simulink model "gm_parallel_prediction_and_cost_function_6phase"  (R2022a)
settings: Solver=FixedStepDiscrete  StartTime=0.0  StopTime=10.0  RelTol=1e-3
undefined symbols (not defined in the file or in its folder): f_c, L_d, L_q, L_x, L_y, p, psi_pm, R_ph
libraries: hdlmdlgenlib x2
(part 3 of 8)

== system gm_parallel_prediction_and_cost_function_6phase/Prediction_and_cost_function/Detect Rise Positive ==
  note: Edge
  note: U(k)
  U : Inport  OutDataTypeStr=boolean  SampleTime=1e-08
  Delay Input1 : UnitDelay  Description=Store in Global RAM  DisableCoverage=on  InitialCondition=vinit  SampleTime=-1  HasFrameUpgradeWarning=on
  FixPt Relational Operator : RelationalOperator  Operator=>  OutDataTypeStr=boolean  ZeroCross=off  InputSameDT=off
  Positive : Subsystem  mask(Compare To Zero){relop=>, OutDataTypeStr=boolean, ZeroCross=off}
      mask prompts: relop "Simulink:masks:Operator_MP"; OutDataTypeStr "Simulink:masks:OutputDataType_MP"; ZeroCross "Simulink:masks:EnableZerocrossingDetection_MP"
      mask help: Simulink:masks:CompareToZero_MD
      mask init:
      | OutDataTypeStr = 'boolean';
      | ZeroCross = 'off';
      | blkName = 'parallel_prediction_and_cost_function_6phase/Prediction_and_cost_function/Detect Rise\nPositive/Positive';
      | relop = '>';
      | setValue = 'boolean';
      mask TypeOptions relop: == | ~= | < | <= | >= | >
      mask TypeOptions OutDataTypeStr: Simulink:masks:uint8 | Simulink:masks:boolean
      mask Callback ZeroCross: sl('zeroCrossEnable', gcbh);
      mask Display: disp([relop,' 0'])
  Y : Outport  SampleTime=1e-08
  wires:
  Delay Input1/1 -> FixPt Relational Operator/2
  FixPt Relational Operator/1 -> Y/1
  Positive/1(y) -> FixPt Relational Operator/1, Delay Input1/1
  U/1 -> Positive/1(u)

== system gm_parallel_prediction_and_cost_function_6phase/Prediction_and_cost_function/Detect Rise Positive1 ==
  note: Edge
  note: U(k)
  U : Inport  OutDataTypeStr=boolean  SampleTime=1e-08
  Delay Input1 : UnitDelay  Description=Store in Global RAM  DisableCoverage=on  InitialCondition=vinit  SampleTime=-1  HasFrameUpgradeWarning=on
  FixPt Relational Operator : RelationalOperator  Operator=>  OutDataTypeStr=boolean  ZeroCross=off  InputSameDT=off
  Positive : Subsystem  mask(Compare To Zero){relop=>, OutDataTypeStr=boolean, ZeroCross=off}
      mask prompts: relop "Simulink:masks:Operator_MP"; OutDataTypeStr "Simulink:masks:OutputDataType_MP"; ZeroCross "Simulink:masks:EnableZerocrossingDetection_MP"
      mask help: Simulink:masks:CompareToZero_MD
      mask init:
      | OutDataTypeStr = 'boolean';
      | ZeroCross = 'off';
      | blkName = 'parallel_prediction_and_cost_function_6phase/Prediction_and_cost_function/Detect Rise\nPositive1/Positive';
      | relop = '>';
      | setValue = 'boolean';
      mask TypeOptions relop: == | ~= | < | <= | >= | >
      mask TypeOptions OutDataTypeStr: Simulink:masks:uint8 | Simulink:masks:boolean
      mask Callback ZeroCross: sl('zeroCrossEnable', gcbh);
      mask Display: disp([relop,' 0'])
  Y : Outport  SampleTime=1e-08
  wires:
  Delay Input1/1 -> FixPt Relational Operator/2
  FixPt Relational Operator/1 -> Y/1
  Positive/1(y) -> FixPt Relational Operator/1, Delay Input1/1
  U/1 -> Positive/1(u)

== system gm_parallel_prediction_and_cost_function_6phase/Prediction_and_cost_function/Detect Rise Positive2 ==
  note: Edge
  note: U(k)
  U : Inport  OutDataTypeStr=boolean  SampleTime=1e-08
  Delay Input1 : UnitDelay  Description=Store in Global RAM  DisableCoverage=on  InitialCondition=vinit  SampleTime=-1  HasFrameUpgradeWarning=on
  FixPt Relational Operator : RelationalOperator  Operator=>  OutDataTypeStr=boolean  ZeroCross=off  InputSameDT=off
  Positive : Subsystem  mask(Compare To Zero){relop=>, OutDataTypeStr=boolean, ZeroCross=off}
      mask prompts: relop "Simulink:masks:Operator_MP"; OutDataTypeStr "Simulink:masks:OutputDataType_MP"; ZeroCross "Simulink:masks:EnableZerocrossingDetection_MP"
      mask help: Simulink:masks:CompareToZero_MD
      mask init:
      | OutDataTypeStr = 'boolean';
      | ZeroCross = 'off';
      | blkName = 'parallel_prediction_and_cost_function_6phase/Prediction_and_cost_function/Detect Rise\nPositive2/Positive';
      | relop = '>';
      | setValue = 'boolean';
      mask TypeOptions relop: == | ~= | < | <= | >= | >
      mask TypeOptions OutDataTypeStr: Simulink:masks:uint8 | Simulink:masks:boolean
      mask Callback ZeroCross: sl('zeroCrossEnable', gcbh);
      mask Display: disp([relop,' 0'])
  Y : Outport  SampleTime=1e-08
  wires:
  Delay Input1/1 -> FixPt Relational Operator/2
  FixPt Relational Operator/1 -> Y/1
  Positive/1(y) -> FixPt Relational Operator/1, Delay Input1/1
  U/1 -> Positive/1(u)

== system gm_parallel_prediction_and_cost_function_6phase/Prediction_and_cost_function/Product ==
  In1 : Inport
  In2 : Inport  Port=2
  Product : Product  Inputs=**  OutDataTypeStr=single  SampleTime=1e-08
  Product_pd1 : Delay  DelayLength=6
  Out1 : Outport
  wires:
  In1/1 -> Product/1
  In2/1 -> Product/2
  Product/1 -> Product_pd1/1
  Product_pd1/1 -> Out1/1

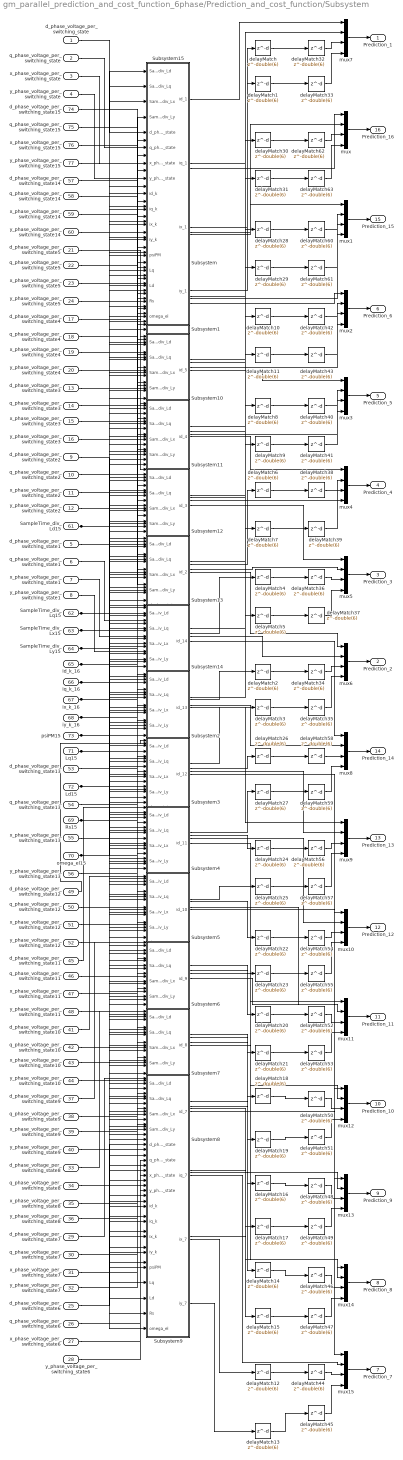
== system gm_parallel_prediction_and_cost_function_6phase/Prediction_and_cost_function/Subsystem ==
  d_phase_voltage_per_switching_state : Inport  OutDataTypeStr=single  PortDimensions=1  SampleTime=1e-08
  q_phase_voltage_per_switching_state : Inport  Port=2  OutDataTypeStr=single  PortDimensions=1  SampleTime=1e-08
  x_phase_voltage_per_switching_state : Inport  Port=3  OutDataTypeStr=single  PortDimensions=1  SampleTime=1e-08
  y_phase_voltage_per_switching_state : Inport  Port=4  OutDataTypeStr=single  PortDimensions=1  SampleTime=1e-08
  d_phase_voltage_per_switching_state1 : Inport  Port=5  OutDataTypeStr=single  PortDimensions=1  SampleTime=1e-08
  q_phase_voltage_per_switching_state1 : Inport  Port=6  OutDataTypeStr=single  PortDimensions=1  SampleTime=1e-08
  x_phase_voltage_per_switching_state1 : Inport  Port=7  OutDataTypeStr=single  PortDimensions=1  SampleTime=1e-08
  y_phase_voltage_per_switching_state1 : Inport  Port=8  OutDataTypeStr=single  PortDimensions=1  SampleTime=1e-08
  d_phase_voltage_per_switching_state2 : Inport  Port=9  OutDataTypeStr=single  PortDimensions=1  SampleTime=1e-08
  q_phase_voltage_per_switching_state2 : Inport  Port=10  OutDataTypeStr=single  PortDimensions=1  SampleTime=1e-08
  x_phase_voltage_per_switching_state2 : Inport  Port=11  OutDataTypeStr=single  PortDimensions=1  SampleTime=1e-08
  y_phase_voltage_per_switching_state2 : Inport  Port=12  OutDataTypeStr=single  PortDimensions=1  SampleTime=1e-08
  d_phase_voltage_per_switching_state3 : Inport  Port=13  OutDataTypeStr=single  PortDimensions=1  SampleTime=1e-08
  q_phase_voltage_per_switching_state3 : Inport  Port=14  OutDataTypeStr=single  PortDimensions=1  SampleTime=1e-08
  x_phase_voltage_per_switching_state3 : Inport  Port=15  OutDataTypeStr=single  PortDimensions=1  SampleTime=1e-08
  y_phase_voltage_per_switching_state3 : Inport  Port=16  OutDataTypeStr=single  PortDimensions=1  SampleTime=1e-08
  d_phase_voltage_per_switching_state4 : Inport  Port=17  OutDataTypeStr=single  PortDimensions=1  SampleTime=1e-08
  q_phase_voltage_per_switching_state4 : Inport  Port=18  OutDataTypeStr=single  PortDimensions=1  SampleTime=1e-08
  x_phase_voltage_per_switching_state4 : Inport  Port=19  OutDataTypeStr=single  PortDimensions=1  SampleTime=1e-08
  y_phase_voltage_per_switching_state4 : Inport  Port=20  OutDataTypeStr=single  PortDimensions=1  SampleTime=1e-08
  d_phase_voltage_per_switching_state5 : Inport  Port=21  OutDataTypeStr=single  PortDimensions=1  SampleTime=1e-08
  q_phase_voltage_per_switching_state5 : Inport  Port=22  OutDataTypeStr=single  PortDimensions=1  SampleTime=1e-08
  x_phase_voltage_per_switching_state5 : Inport  Port=23  OutDataTypeStr=single  PortDimensions=1  SampleTime=1e-08
  y_phase_voltage_per_switching_state5 : Inport  Port=24  OutDataTypeStr=single  PortDimensions=1  SampleTime=1e-08
  d_phase_voltage_per_switching_state6 : Inport  Port=25  OutDataTypeStr=single  PortDimensions=1  SampleTime=1e-08
  q_phase_voltage_per_switching_state6 : Inport  Port=26  OutDataTypeStr=single  PortDimensions=1  SampleTime=1e-08
  x_phase_voltage_per_switching_state6 : Inport  Port=27  OutDataTypeStr=single  PortDimensions=1  SampleTime=1e-08
  y_phase_voltage_per_switching_state6 : Inport  Port=28  OutDataTypeStr=single  PortDimensions=1  SampleTime=1e-08
  d_phase_voltage_per_switching_state7 : Inport  Port=29  OutDataTypeStr=single  PortDimensions=1  SampleTime=1e-08
  q_phase_voltage_per_switching_state7 : Inport  Port=30  OutDataTypeStr=single  PortDimensions=1  SampleTime=1e-08
  x_phase_voltage_per_switching_state7 : Inport  Port=31  OutDataTypeStr=single  PortDimensions=1  SampleTime=1e-08
  y_phase_voltage_per_switching_state7 : Inport  Port=32  OutDataTypeStr=single  PortDimensions=1  SampleTime=1e-08
  d_phase_voltage_per_switching_state8 : Inport  Port=33  OutDataTypeStr=single  PortDimensions=1  SampleTime=1e-08
  q_phase_voltage_per_switching_state8 : Inport  Port=34  OutDataTypeStr=single  PortDimensions=1  SampleTime=1e-08
  x_phase_voltage_per_switching_state8 : Inport  Port=35  OutDataTypeStr=single  PortDimensions=1  SampleTime=1e-08
  y_phase_voltage_per_switching_state8 : Inport  Port=36  OutDataTypeStr=single  PortDimensions=1  SampleTime=1e-08
  d_phase_voltage_per_switching_state9 : Inport  Port=37  OutDataTypeStr=single  PortDimensions=1  SampleTime=1e-08
  q_phase_voltage_per_switching_state9 : Inport  Port=38  OutDataTypeStr=single  PortDimensions=1  SampleTime=1e-08
  x_phase_voltage_per_switching_state9 : Inport  Port=39  OutDataTypeStr=single  PortDimensions=1  SampleTime=1e-08
  y_phase_voltage_per_switching_state9 : Inport  Port=40  OutDataTypeStr=single  PortDimensions=1  SampleTime=1e-08
  d_phase_voltage_per_switching_state10 : Inport  Port=41  OutDataTypeStr=single  PortDimensions=1  SampleTime=1e-08
  q_phase_voltage_per_switching_state10 : Inport  Port=42  OutDataTypeStr=single  PortDimensions=1  SampleTime=1e-08
  x_phase_voltage_per_switching_state10 : Inport  Port=43  OutDataTypeStr=single  PortDimensions=1  SampleTime=1e-08
  y_phase_voltage_per_switching_state10 : Inport  Port=44  OutDataTypeStr=single  PortDimensions=1  SampleTime=1e-08
  d_phase_voltage_per_switching_state11 : Inport  Port=45  OutDataTypeStr=single  PortDimensions=1  SampleTime=1e-08
  q_phase_voltage_per_switching_state11 : Inport  Port=46  OutDataTypeStr=single  PortDimensions=1  SampleTime=1e-08
  x_phase_voltage_per_switching_state11 : Inport  Port=47  OutDataTypeStr=single  PortDimensions=1  SampleTime=1e-08
  y_phase_voltage_per_switching_state11 : Inport  Port=48  OutDataTypeStr=single  PortDimensions=1  SampleTime=1e-08
  d_phase_voltage_per_switching_state12 : Inport  Port=49  OutDataTypeStr=single  PortDimensions=1  SampleTime=1e-08
  q_phase_voltage_per_switching_state12 : Inport  Port=50  OutDataTypeStr=single  PortDimensions=1  SampleTime=1e-08
  x_phase_voltage_per_switching_state12 : Inport  Port=51  OutDataTypeStr=single  PortDimensions=1  SampleTime=1e-08
  y_phase_voltage_per_switching_state12 : Inport  Port=52  OutDataTypeStr=single  PortDimensions=1  SampleTime=1e-08
  d_phase_voltage_per_switching_state13 : Inport  Port=53  OutDataTypeStr=single  PortDimensions=1  SampleTime=1e-08
  q_phase_voltage_per_switching_state13 : Inport  Port=54  OutDataTypeStr=single  PortDimensions=1  SampleTime=1e-08
  x_phase_voltage_per_switching_state13 : Inport  Port=55  OutDataTypeStr=single  PortDimensions=1  SampleTime=1e-08
  y_phase_voltage_per_switching_state13 : Inport  Port=56  OutDataTypeStr=single  PortDimensions=1  SampleTime=1e-08
  d_phase_voltage_per_switching_state14 : Inport  Port=57  OutDataTypeStr=single  PortDimensions=1  SampleTime=1e-08
  q_phase_voltage_per_switching_state14 : Inport  Port=58  OutDataTypeStr=single  PortDimensions=1  SampleTime=1e-08
  x_phase_voltage_per_switching_state14 : Inport  Port=59  OutDataTypeStr=single  PortDimensions=1  SampleTime=1e-08
  y_phase_voltage_per_switching_state14 : Inport  Port=60  OutDataTypeStr=single  PortDimensions=1  SampleTime=1e-08
  SampleTime_div_Ld15 : Inport  Port=61  OutDataTypeStr=single  PortDimensions=1  SampleTime=1e-08
  SampleTime_div_Lq15 : Inport  Port=62  OutDataTypeStr=single  PortDimensions=1  SampleTime=1e-08
  SampleTime_div_Lx15 : Inport  Port=63  OutDataTypeStr=single  PortDimensions=1  SampleTime=1e-08
  SampleTime_div_Ly15 : Inport  Port=64  OutDataTypeStr=single  PortDimensions=1  SampleTime=1e-08
  id_k_16 : Inport  Port=65  OutDataTypeStr=single  PortDimensions=1  SampleTime=1e-08
  iq_k_16 : Inport  Port=66  OutDataTypeStr=single  PortDimensions=1  SampleTime=1e-08
  ix_k_16 : Inport  Port=67  OutDataTypeStr=single  PortDimensions=1  SampleTime=1e-08
  iy_k_16 : Inport  Port=68  OutDataTypeStr=single  PortDimensions=1  SampleTime=1e-08
  Rs15 : Inport  Port=69  OutDataTypeStr=single  PortDimensions=1  SampleTime=1e-08
  omega_el15 : Inport  Port=70  OutDataTypeStr=single  PortDimensions=1  SampleTime=1e-08
  Lq15 : Inport  Port=71  OutDataTypeStr=single  PortDimensions=1  SampleTime=1e-08
  Ld15 : Inport  Port=72  OutDataTypeStr=single  PortDimensions=1  SampleTime=1e-08
  psiPM15 : Inport  Port=73  OutDataTypeStr=single  PortDimensions=1  SampleTime=1e-08
  d_phase_voltage_per_switching_state15 : Inport  Port=74  OutDataTypeStr=single  PortDimensions=1  SampleTime=1e-08
  q_phase_voltage_per_switching_state15 : Inport  Port=75  OutDataTypeStr=single  PortDimensions=1  SampleTime=1e-08
  x_phase_voltage_per_switching_state15 : Inport  Port=76  OutDataTypeStr=single  PortDimensions=1  SampleTime=1e-08
  y_phase_voltage_per_switching_state15 : Inport  Port=77  OutDataTypeStr=single  PortDimensions=1  SampleTime=1e-08
  Subsystem : Subsystem
  Subsystem1 : Subsystem
  Subsystem10 : Subsystem
  Subsystem11 : Subsystem
  Subsystem12 : Subsystem
  Subsystem13 : Subsystem
  Subsystem14 : Subsystem
  Subsystem15 : Subsystem
  Subsystem2 : Subsystem
  Subsystem3 : Subsystem
  Subsystem4 : Subsystem
  Subsystem5 : Subsystem
  Subsystem6 : Subsystem
  Subsystem7 : Subsystem
  Subsystem8 : Subsystem
  Subsystem9 : Subsystem
  delayMatch{,1..63} (64 alike) : Delay  DelayLength=double(6)  InitialCondition=0  SampleTime=1e-08
  mux{,1..15} (16 alike) : Mux
  Prediction_1 : Outport  SampleTime=1e-08
  Prediction_2 : Outport  Port=2  SampleTime=1e-08
  Prediction_3 : Outport  Port=3  SampleTime=1e-08
  Prediction_4 : Outport  Port=4  SampleTime=1e-08
  Prediction_5 : Outport  Port=5  SampleTime=1e-08
  Prediction_6 : Outport  Port=6  SampleTime=1e-08
  Prediction_7 : Outport  Port=7  SampleTime=1e-08
  Prediction_8 : Outport  Port=8  SampleTime=1e-08
  Prediction_9 : Outport  Port=9  SampleTime=1e-08
  Prediction_10 : Outport  Port=10  SampleTime=1e-08
  Prediction_11 : Outport  Port=11  SampleTime=1e-08
  Prediction_12 : Outport  Port=12  SampleTime=1e-08
  Prediction_13 : Outport  Port=13  SampleTime=1e-08
  Prediction_14 : Outport  Port=14  SampleTime=1e-08
  Prediction_15 : Outport  Port=15  SampleTime=1e-08
  Prediction_16 : Outport  Port=16  SampleTime=1e-08
  wires:
  mux/1 -> Prediction_16/1
  mux1/1 -> Prediction_15/1
  mux2/1 -> Prediction_6/1
  mux3/1 -> Prediction_5/1
  mux4/1 -> Prediction_4/1
  mux5/1 -> Prediction_3/1
  mux6/1 -> Prediction_2/1
  mux7/1 -> Prediction_1/1
  mux8/1 -> Prediction_14/1
  mux9/1 -> Prediction_13/1
  mux10/1 -> Prediction_12/1
  mux11/1 -> Prediction_11/1
  mux12/1 -> Prediction_10/1
  mux13/1 -> Prediction_9/1
  mux14/1 -> Prediction_8/1
  mux15/1 -> Prediction_7/1
  Subsystem/2(iq_16) -> mux/2
  delayMatch62/1 -> mux/3
  delayMatch63/1 -> mux/4
  Subsystem1/2(iq_15) -> mux1/2
  delayMatch60/1 -> mux1/3
  delayMatch61/1 -> mux1/4
  Subsystem10/2(iq_6) -> mux2/2
  delayMatch42/1 -> mux2/3
  delayMatch43/1 -> mux2/4
  Subsystem11/2(iq_5) -> mux3/2
  delayMatch40/1 -> mux3/3
  delayMatch41/1 -> mux3/4
  Subsystem12/2(iq_4) -> mux4/2
  delayMatch38/1 -> mux4/3
  delayMatch39/1 -> mux4/4
  Subsystem13/2(iq_3) -> mux5/2
  delayMatch36/1 -> mux5/3
  delayMatch37/1 -> mux5/4
  Subsystem14/2(iq_2) -> mux6/2
  delayMatch34/1 -> mux6/3
  delayMatch35/1 -> mux6/4
  Subsystem15/2(iq_1) -> mux7/2
  delayMatch32/1 -> mux7/3
  delayMatch33/1 -> mux7/4
  Subsystem2/2(iq_14) -> mux8/2
  delayMatch58/1 -> mux8/3
  delayMatch59/1 -> mux8/4
  Subsystem3/2(iq_13) -> mux9/2
  delayMatch56/1 -> mux9/3
  delayMatch57/1 -> mux9/4
  Subsystem4/2(iq_12) -> mux10/2
  delayMatch54/1 -> mux10/3
  delayMatch55/1 -> mux10/4
  Subsystem5/2(iq_11) -> mux11/2
  delayMatch52/1 -> mux11/3
  delayMatch53/1 -> mux11/4
  Subsystem6/2(iq_10) -> mux12/2
  delayMatch50/1 -> mux12/3
  delayMatch51/1 -> mux12/4
  Subsystem7/2(iq_9) -> mux13/2
  delayMatch48/1 -> mux13/3
  delayMatch49/1 -> mux13/4
  Subsystem8/2(iq_8) -> mux14/2
  delayMatch46/1 -> mux14/3
  delayMatch47/1 -> mux14/4
  Subsystem9/2(iq_7) -> mux15/2
  delayMatch44/1 -> mux15/3
  delayMatch45/1 -> mux15/4
  Subsystem15/1(id_1) -> mux7/1
  Subsystem15/3(ix_1) -> delayMatch/1
  Subsystem15/4(iy_1) -> delayMatch1/1
  Subsystem14/1(id_2) -> mux6/1
  Subsystem14/3(ix_2) -> delayMatch2/1
  Subsystem14/4(iy_2) -> delayMatch3/1
  Subsystem13/1(id_3) -> mux5/1
  Subsystem13/3(ix_3) -> delayMatch4/1
  Subsystem13/4(iy_3) -> delayMatch5/1
  Subsystem12/1(id_4) -> mux4/1
  Subsystem12/3(ix_4) -> delayMatch6/1
  Subsystem12/4(iy_4) -> delayMatch7/1
  Subsystem11/1(id_5) -> mux3/1
  Subsystem11/3(ix_5) -> delayMatch8/1
  Subsystem11/4(iy_5) -> delayMatch9/1
  Subsystem10/1(id_6) -> mux2/1
  Subsystem10/3(ix_6) -> delayMatch10/1
  Subsystem10/4(iy_6) -> delayMatch11/1
  Subsystem9/1(id_7) -> mux15/1
  Subsystem9/3(ix_7) -> delayMatch12/1
  Subsystem9/4(iy_7) -> delayMatch13/1
  Subsystem8/1(id_8) -> mux14/1
  Subsystem8/3(ix_8) -> delayMatch14/1
  Subsystem8/4(iy_8) -> delayMatch15/1
  Subsystem7/1(id_9) -> mux13/1
  Subsystem7/3(ix_9) -> delayMatch16/1
  Subsystem7/4(iy_9) -> delayMatch17/1
  Subsystem6/1(id_10) -> mux12/1
  Subsystem6/3(ix_10) -> delayMatch18/1
  Subsystem6/4(iy_10) -> delayMatch19/1
  Subsystem5/1(id_11) -> mux11/1
  Subsystem5/3(ix_11) -> delayMatch20/1
  Subsystem5/4(iy_11) -> delayMatch21/1
  Subsystem4/1(id_12) -> mux10/1
  Subsystem4/3(ix_12) -> delayMatch22/1
  Subsystem4/4(iy_12) -> delayMatch23/1
  Subsystem3/1(id_13) -> mux9/1
  Subsystem3/3(ix_13) -> delayMatch24/1
  Subsystem3/4(iy_13) -> delayMatch25/1
  Subsystem2/1(id_14) -> mux8/1
  Subsystem2/3(ix_14) -> delayMatch26/1
  Subsystem2/4(iy_14) -> delayMatch27/1
  Subsystem1/1(id_15) -> mux1/1
  Subsystem1/3(ix_15) -> delayMatch28/1
  Subsystem1/4(iy_15) -> delayMatch29/1
  Subsystem/1(id_16) -> mux/1
  Subsystem/3(ix_16) -> delayMatch30/1
  Subsystem/4(iy_16) -> delayMatch31/1
  delayMatch/1 -> delayMatch32/1
  delayMatch1/1 -> delayMatch33/1
  delayMatch2/1 -> delayMatch34/1
  delayMatch3/1 -> delayMatch35/1
  delayMatch4/1 -> delayMatch36/1
  delayMatch5/1 -> delayMatch37/1
  delayMatch6/1 -> delayMatch38/1
  delayMatch7/1 -> delayMatch39/1
  delayMatch8/1 -> delayMatch40/1
  delayMatch9/1 -> delayMatch41/1
  delayMatch10/1 -> delayMatch42/1
  delayMatch11/1 -> delayMatch43/1
  delayMatch12/1 -> delayMatch44/1
  delayMatch13/1 -> delayMatch45/1
  delayMatch14/1 -> delayMatch46/1
  delayMatch15/1 -> delayMatch47/1
  delayMatch16/1 -> delayMatch48/1
  delayMatch17/1 -> delayMatch49/1
  delayMatch18/1 -> delayMatch50/1
  delayMatch19/1 -> delayMatch51/1
  delayMatch20/1 -> delayMatch52/1
  delayMatch21/1 -> delayMatch53/1
  delayMatch22/1 -> delayMatch54/1
  delayMatch23/1 -> delayMatch55/1
  delayMatch24/1 -> delayMatch56/1
  delayMatch25/1 -> delayMatch57/1
  delayMatch26/1 -> delayMatch58/1
  delayMatch27/1 -> delayMatch59/1
  delayMatch28/1 -> delayMatch60/1
  delayMatch29/1 -> delayMatch61/1
  delayMatch30/1 -> delayMatch62/1
  delayMatch31/1 -> delayMatch63/1
  d_phase_voltage_per_switching_state/1 -> Subsystem15/5(d_phase_voltage_per_switching_state)
  q_phase_voltage_per_switching_state/1 -> Subsystem15/6(q_phase_voltage_per_switching_state)
  x_phase_voltage_per_switching_state/1 -> Subsystem15/7(x_phase_voltage_per_switching_state)
  y_phase_voltage_per_switching_state/1 -> Subsystem15/8(y_phase_voltage_per_switching_state)
  d_phase_voltage_per_switching_state1/1 -> Subsystem14/5(d_phase_voltage_per_switching_state)
  q_phase_voltage_per_switching_state1/1 -> Subsystem14/6(q_phase_voltage_per_switching_state)
  x_phase_voltage_per_switching_state1/1 -> Subsystem14/7(x_phase_voltage_per_switching_state)
  y_phase_voltage_per_switching_state1/1 -> Subsystem14/8(y_phase_voltage_per_switching_state)
  d_phase_voltage_per_switching_state2/1 -> Subsystem13/5(d_phase_voltage_per_switching_state)
  q_phase_voltage_per_switching_state2/1 -> Subsystem13/6(q_phase_voltage_per_switching_state)
  x_phase_voltage_per_switching_state2/1 -> Subsystem13/7(x_phase_voltage_per_switching_state)
  y_phase_voltage_per_switching_state2/1 -> Subsystem13/8(y_phase_voltage_per_switching_state)
  d_phase_voltage_per_switching_state3/1 -> Subsystem12/5(d_phase_voltage_per_switching_state)
  q_phase_voltage_per_switching_state3/1 -> Subsystem12/6(q_phase_voltage_per_switching_state)
  x_phase_voltage_per_switching_state3/1 -> Subsystem12/7(x_phase_voltage_per_switching_state)
  y_phase_voltage_per_switching_state3/1 -> Subsystem12/8(y_phase_voltage_per_switching_state)
  d_phase_voltage_per_switching_state4/1 -> Subsystem11/5(d_phase_voltage_per_switching_state)
  q_phase_voltage_per_switching_state4/1 -> Subsystem11/6(q_phase_voltage_per_switching_state)
  x_phase_voltage_per_switching_state4/1 -> Subsystem11/7(x_phase_voltage_per_switching_state)
  y_phase_voltage_per_switching_state4/1 -> Subsystem11/8(y_phase_voltage_per_switching_state)
  d_phase_voltage_per_switching_state5/1 -> Subsystem10/5(d_phase_voltage_per_switching_state)
  q_phase_voltage_per_switching_state5/1 -> Subsystem10/6(q_phase_voltage_per_switching_state)
  x_phase_voltage_per_switching_state5/1 -> Subsystem10/7(x_phase_voltage_per_switching_state)
  y_phase_voltage_per_switching_state5/1 -> Subsystem10/8(y_phase_voltage_per_switching_state)
  d_phase_voltage_per_switching_state6/1 -> Subsystem9/5(d_phase_voltage_per_switching_state)
  q_phase_voltage_per_switching_state6/1 -> Subsystem9/6(q_phase_voltage_per_switching_state)
  x_phase_voltage_per_switching_state6/1 -> Subsystem9/7(x_phase_voltage_per_switching_state)
  y_phase_voltage_per_switching_state6/1 -> Subsystem9/8(y_phase_voltage_per_switching_state)
  d_phase_voltage_per_switching_state7/1 -> Subsystem8/5(d_phase_voltage_per_switching_state)
  q_phase_voltage_per_switching_state7/1 -> Subsystem8/6(q_phase_voltage_per_switching_state)
  x_phase_voltage_per_switching_state7/1 -> Subsystem8/7(x_phase_voltage_per_switching_state)
  y_phase_voltage_per_switching_state7/1 -> Subsystem8/8(y_phase_voltage_per_switching_state)
  d_phase_voltage_per_switching_state8/1 -> Subsystem7/5(d_phase_voltage_per_switching_state)
  q_phase_voltage_per_switching_state8/1 -> Subsystem7/6(q_phase_voltage_per_switching_state)
  x_phase_voltage_per_switching_state8/1 -> Subsystem7/7(x_phase_voltage_per_switching_state)
  y_phase_voltage_per_switching_state8/1 -> Subsystem7/8(y_phase_voltage_per_switching_state)
  d_phase_voltage_per_switching_state9/1 -> Subsystem6/5(d_phase_voltage_per_switching_state)
  q_phase_voltage_per_switching_state9/1 -> Subsystem6/6(q_phase_voltage_per_switching_state)
  x_phase_voltage_per_switching_state9/1 -> Subsystem6/7(x_phase_voltage_per_switching_state)
  y_phase_voltage_per_switching_state9/1 -> Subsystem6/8(y_phase_voltage_per_switching_state)
  d_phase_voltage_per_switching_state10/1 -> Subsystem5/5(d_phase_voltage_per_switching_state)
  q_phase_voltage_per_switching_state10/1 -> Subsystem5/6(q_phase_voltage_per_switching_state)
  x_phase_voltage_per_switching_state10/1 -> Subsystem5/7(x_phase_voltage_per_switching_state)
  y_phase_voltage_per_switching_state10/1 -> Subsystem5/8(y_phase_voltage_per_switching_state)
  d_phase_voltage_per_switching_state11/1 -> Subsystem4/5(d_phase_voltage_per_switching_state)
  q_phase_voltage_per_switching_state11/1 -> Subsystem4/6(q_phase_voltage_per_switching_state)
  x_phase_voltage_per_switching_state11/1 -> Subsystem4/7(x_phase_voltage_per_switching_state)
  y_phase_voltage_per_switching_state11/1 -> Subsystem4/8(y_phase_voltage_per_switching_state)
  d_phase_voltage_per_switching_state12/1 -> Subsystem3/5(d_phase_voltage_per_switching_state)
  q_phase_voltage_per_switching_state12/1 -> Subsystem3/6(q_phase_voltage_per_switching_state)
  x_phase_voltage_per_switching_state12/1 -> Subsystem3/7(x_phase_voltage_per_switching_state)
  y_phase_voltage_per_switching_state12/1 -> Subsystem3/8(y_phase_voltage_per_switching_state)
  d_phase_voltage_per_switching_state13/1 -> Subsystem2/5(d_phase_voltage_per_switching_state)
  q_phase_voltage_per_switching_state13/1 -> Subsystem2/6(q_phase_voltage_per_switching_state)
  x_phase_voltage_per_switching_state13/1 -> Subsystem2/7(x_phase_voltage_per_switching_state)
  y_phase_voltage_per_switching_state13/1 -> Subsystem2/8(y_phase_voltage_per_switching_state)
  d_phase_voltage_per_switching_state14/1 -> Subsystem1/5(d_phase_voltage_per_switching_state)
  q_phase_voltage_per_switching_state14/1 -> Subsystem1/6(q_phase_voltage_per_switching_state)
  x_phase_voltage_per_switching_state14/1 -> Subsystem1/7(x_phase_voltage_per_switching_state)
  y_phase_voltage_per_switching_state14/1 -> Subsystem1/8(y_phase_voltage_per_switching_state)
  SampleTime_div_Ld15/1 -> Subsystem/1(SampleTime_div_Ld), Subsystem4/1(SampleTime_div_Ld), Subsystem7/1(SampleTime_div_Ld), Subsystem15/1(SampleTime_div_Ld), Subsystem14/1(SampleTime_div_Ld), Subsystem13/1(SampleTime_div_Ld), Subsystem12/1(SampleTime_div_Ld), Subsystem11/1(SampleTime_div_Ld), Subsystem10/1(SampleTime_div_Ld), Subsystem9/1(SampleTime_div_Ld), Subsystem8/1(SampleTime_div_Ld), Subsystem6/1(SampleTime_div_Ld), Subsystem5/1(SampleTime_div_Ld), Subsystem3/1(SampleTime_div_Ld), Subsystem2/1(SampleTime_div_Ld), Subsystem1/1(SampleTime_div_Ld)
  SampleTime_div_Lq15/1 -> Subsystem/2(SampleTime_div_Lq), Subsystem4/2(SampleTime_div_Lq), Subsystem15/2(SampleTime_div_Lq), Subsystem14/2(SampleTime_div_Lq), Subsystem13/2(SampleTime_div_Lq), Subsystem12/2(SampleTime_div_Lq), Subsystem11/2(SampleTime_div_Lq), Subsystem10/2(SampleTime_div_Lq), Subsystem9/2(SampleTime_div_Lq), Subsystem8/2(SampleTime_div_Lq), Subsystem7/2(SampleTime_div_Lq), Subsystem6/2(SampleTime_div_Lq), Subsystem5/2(SampleTime_div_Lq), Subsystem3/2(SampleTime_div_Lq), Subsystem2/2(SampleTime_div_Lq), Subsystem1/2(SampleTime_div_Lq)
  SampleTime_div_Lx15/1 -> Subsystem/3(SampleTime_div_Lx), Subsystem15/3(SampleTime_div_Lx), Subsystem14/3(SampleTime_div_Lx), Subsystem13/3(SampleTime_div_Lx), Subsystem12/3(SampleTime_div_Lx), Subsystem11/3(SampleTime_div_Lx), Subsystem10/3(SampleTime_div_Lx), Subsystem9/3(SampleTime_div_Lx), Subsystem8/3(SampleTime_div_Lx), Subsystem7/3(SampleTime_div_Lx), Subsystem6/3(SampleTime_div_Lx), Subsystem5/3(SampleTime_div_Lx), Subsystem4/3(SampleTime_div_Lx), Subsystem3/3(SampleTime_div_Lx), Subsystem2/3(SampleTime_div_Lx), Subsystem1/3(SampleTime_div_Lx)
  SampleTime_div_Ly15/1 -> Subsystem15/4(SampleTime_div_Ly), Subsystem14/4(SampleTime_div_Ly), Subsystem13/4(SampleTime_div_Ly), Subsystem12/4(SampleTime_div_Ly), Subsystem11/4(SampleTime_div_Ly), Subsystem10/4(SampleTime_div_Ly), Subsystem9/4(SampleTime_div_Ly), Subsystem8/4(SampleTime_div_Ly), Subsystem7/4(SampleTime_div_Ly), Subsystem6/4(SampleTime_div_Ly), Subsystem5/4(SampleTime_div_Ly), Subsystem4/4(SampleTime_div_Ly), Subsystem3/4(SampleTime_div_Ly), Subsystem2/4(SampleTime_div_Ly), Subsystem1/4(SampleTime_div_Ly), Subsystem/4(SampleTime_div_Ly)
  id_k_16/1 -> Subsystem/9(id_k), Subsystem15/9(id_k), Subsystem14/9(id_k), Subsystem13/9(id_k), Subsystem12/9(id_k), Subsystem11/9(id_k), Subsystem10/9(id_k), Subsystem9/9(id_k), Subsystem8/9(id_k), Subsystem7/9(id_k), Subsystem6/9(id_k), Subsystem5/9(id_k), Subsystem4/9(id_k), Subsystem3/9(id_k), Subsystem2/9(id_k), Subsystem1/9(id_k)
  iq_k_16/1 -> Subsystem/10(iq_k), Subsystem15/10(iq_k), Subsystem14/10(iq_k), Subsystem13/10(iq_k), Subsystem12/10(iq_k), Subsystem11/10(iq_k), Subsystem10/10(iq_k), Subsystem9/10(iq_k), Subsystem8/10(iq_k), Subsystem7/10(iq_k), Subsystem6/10(iq_k), Subsystem5/10(iq_k), Subsystem4/10(iq_k), Subsystem3/10(iq_k), Subsystem2/10(iq_k), Subsystem1/10(iq_k)
  ix_k_16/1 -> Subsystem/11(ix_k), Subsystem15/11(ix_k), Subsystem14/11(ix_k), Subsystem13/11(ix_k), Subsystem12/11(ix_k), Subsystem11/11(ix_k), Subsystem10/11(ix_k), Subsystem9/11(ix_k), Subsystem8/11(ix_k), Subsystem7/11(ix_k), Subsystem6/11(ix_k), Subsystem5/11(ix_k), Subsystem4/11(ix_k), Subsystem3/11(ix_k), Subsystem2/11(ix_k), Subsystem1/11(ix_k)
  iy_k_16/1 -> Subsystem/12(iy_k), Subsystem15/12(iy_k), Subsystem14/12(iy_k), Subsystem13/12(iy_k), Subsystem12/12(iy_k), Subsystem11/12(iy_k), Subsystem10/12(iy_k), Subsystem9/12(iy_k), Subsystem8/12(iy_k), Subsystem7/12(iy_k), Subsystem6/12(iy_k), Subsystem5/12(iy_k), Subsystem4/12(iy_k), Subsystem3/12(iy_k), Subsystem2/12(iy_k), Subsystem1/12(iy_k)
  Rs15/1 -> Subsystem/16(Rs), Subsystem7/16(Rs), Subsystem15/16(Rs), Subsystem14/16(Rs), Subsystem13/16(Rs), Subsystem12/16(Rs), Subsystem11/16(Rs), Subsystem10/16(Rs), Subsystem9/16(Rs), Subsystem8/16(Rs), Subsystem6/16(Rs), Subsystem5/16(Rs), Subsystem4/16(Rs), Subsystem3/16(Rs), Subsystem2/16(Rs), Subsystem1/16(Rs)
  omega_el15/1 -> Subsystem/17(omega_el), Subsystem15/17(omega_el), Subsystem14/17(omega_el), Subsystem13/17(omega_el), Subsystem12/17(omega_el), Subsystem11/17(omega_el), Subsystem10/17(omega_el), Subsystem9/17(omega_el), Subsystem8/17(omega_el), Subsystem7/17(omega_el), Subsystem6/17(omega_el), Subsystem5/17(omega_el), Subsystem4/17(omega_el), Subsystem3/17(omega_el), Subsystem2/17(omega_el), Subsystem1/17(omega_el)
  Lq15/1 -> Subsystem/14(Lq), Subsystem15/14(Lq), Subsystem14/14(Lq), Subsystem13/14(Lq), Subsystem12/14(Lq), Subsystem11/14(Lq), Subsystem10/14(Lq), Subsystem9/14(Lq), Subsystem8/14(Lq), Subsystem7/14(Lq), Subsystem6/14(Lq), Subsystem5/14(Lq), Subsystem4/14(Lq), Subsystem3/14(Lq), Subsystem2/14(Lq), Subsystem1/14(Lq)
  Ld15/1 -> Subsystem/15(Ld), Subsystem1/15(Ld), Subsystem15/15(Ld), Subsystem14/15(Ld), Subsystem13/15(Ld), Subsystem12/15(Ld), Subsystem11/15(Ld), Subsystem10/15(Ld), Subsystem9/15(Ld), Subsystem8/15(Ld), Subsystem7/15(Ld), Subsystem6/15(Ld), Subsystem5/15(Ld), Subsystem4/15(Ld), Subsystem3/15(Ld), Subsystem2/15(Ld)
  psiPM15/1 -> Subsystem/13(psiPM), Subsystem10/13(psiPM), Subsystem15/13(psiPM), Subsystem14/13(psiPM), Subsystem13/13(psiPM), Subsystem12/13(psiPM), Subsystem11/13(psiPM), Subsystem9/13(psiPM), Subsystem8/13(psiPM), Subsystem7/13(psiPM), Subsystem6/13(psiPM), Subsystem5/13(psiPM), Subsystem4/13(psiPM), Subsystem3/13(psiPM), Subsystem2/13(psiPM), Subsystem1/13(psiPM)
  d_phase_voltage_per_switching_state15/1 -> Subsystem/5(d_phase_voltage_per_switching_state)
  q_phase_voltage_per_switching_state15/1 -> Subsystem/6(q_phase_voltage_per_switching_state)
  x_phase_voltage_per_switching_state15/1 -> Subsystem/7(x_phase_voltage_per_switching_state)
  y_phase_voltage_per_switching_state15/1 -> Subsystem/8(y_phase_voltage_per_switching_state)

== system gm_parallel_prediction_and_cost_function_6phase/Prediction_and_cost_function/Detect Rise Positive/Positive ==
  u : Inport  OutDataTypeStr=boolean  SampleTime=1e-08
  Compare : RelationalOperator  Operator=>  OutDataTypeStr=boolean  ZeroCross=off
  Constant : Constant  DisableCoverage=on  Value=0  OutDataTypeStr=Inherit: Inherit via back propagation  SampleTime=-1  PreserveConstantTs=on
  y : Outport  SampleTime=1e-08
  wires:
  Compare/1 -> y/1
  Constant/1 -> Compare/2
  u/1 -> Compare/1

== system gm_parallel_prediction_and_cost_function_6phase/Prediction_and_cost_function/Detect Rise Positive1/Positive ==
  u : Inport  OutDataTypeStr=boolean  SampleTime=1e-08
  Compare : RelationalOperator  Operator=>  OutDataTypeStr=boolean  ZeroCross=off
  Constant : Constant  DisableCoverage=on  Value=0  OutDataTypeStr=Inherit: Inherit via back propagation  SampleTime=-1  PreserveConstantTs=on
  y : Outport  SampleTime=1e-08
  wires:
  Compare/1 -> y/1
  Constant/1 -> Compare/2
  u/1 -> Compare/1

== system gm_parallel_prediction_and_cost_function_6phase/Prediction_and_cost_function/Detect Rise Positive2/Positive ==
  u : Inport  OutDataTypeStr=boolean  SampleTime=1e-08
  Compare : RelationalOperator  Operator=>  OutDataTypeStr=boolean  ZeroCross=off
  Constant : Constant  DisableCoverage=on  Value=0  OutDataTypeStr=Inherit: Inherit via back propagation  SampleTime=-1  PreserveConstantTs=on
  y : Outport  SampleTime=1e-08
  wires:
  Compare/1 -> y/1
  Constant/1 -> Compare/2
  u/1 -> Compare/1

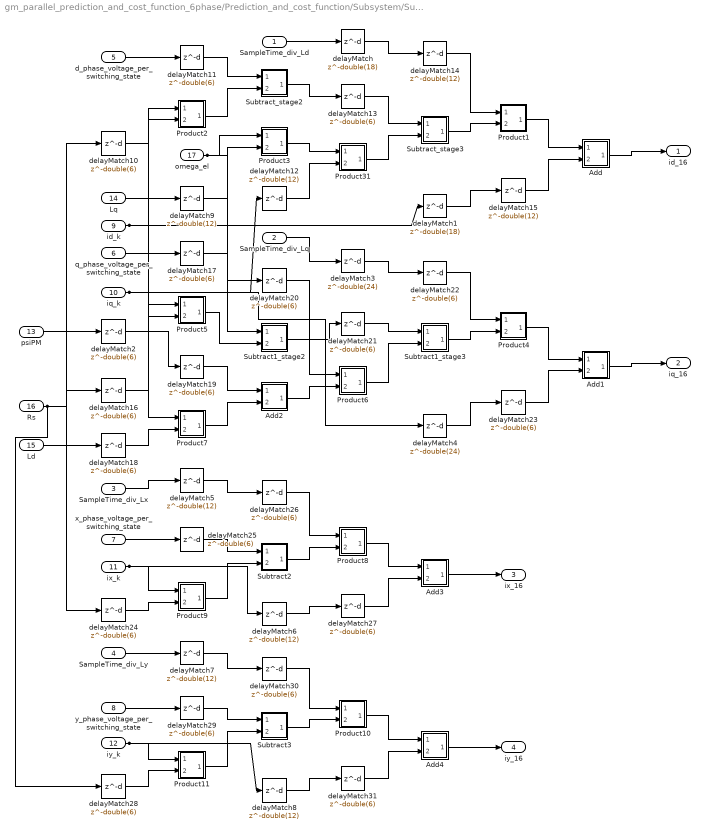
== system gm_parallel_prediction_and_cost_function_6phase/Prediction_and_cost_function/Subsystem/Subsystem ==
  SampleTime_div_Ld : Inport  OutDataTypeStr=single  PortDimensions=1  SampleTime=1e-08
  SampleTime_div_Lq : Inport  Port=2  OutDataTypeStr=single  PortDimensions=1  SampleTime=1e-08
  SampleTime_div_Lx : Inport  Port=3  OutDataTypeStr=single  PortDimensions=1  SampleTime=1e-08
  SampleTime_div_Ly : Inport  Port=4  OutDataTypeStr=single  PortDimensions=1  SampleTime=1e-08
  d_phase_voltage_per_switching_state : Inport  Port=5  OutDataTypeStr=single  PortDimensions=1  SampleTime=1e-08
  q_phase_voltage_per_switching_state : Inport  Port=6  OutDataTypeStr=single  PortDimensions=1  SampleTime=1e-08
  x_phase_voltage_per_switching_state : Inport  Port=7  OutDataTypeStr=single  PortDimensions=1  SampleTime=1e-08
  y_phase_voltage_per_switching_state : Inport  Port=8  OutDataTypeStr=single  PortDimensions=1  SampleTime=1e-08
  id_k : Inport  Port=9  OutDataTypeStr=single  PortDimensions=1  SampleTime=1e-08
  iq_k : Inport  Port=10  OutDataTypeStr=single  PortDimensions=1  SampleTime=1e-08
  ix_k : Inport  Port=11  OutDataTypeStr=single  PortDimensions=1  SampleTime=1e-08
  iy_k : Inport  Port=12  OutDataTypeStr=single  PortDimensions=1  SampleTime=1e-08
  psiPM : Inport  Port=13  OutDataTypeStr=single  PortDimensions=1  SampleTime=1e-08
  Lq : Inport  Port=14  OutDataTypeStr=single  PortDimensions=1  SampleTime=1e-08
  Ld : Inport  Port=15  OutDataTypeStr=single  PortDimensions=1  SampleTime=1e-08
  Rs : Inport  Port=16  OutDataTypeStr=single  PortDimensions=1  SampleTime=1e-08
  omega_el : Inport  Port=17  OutDataTypeStr=single  PortDimensions=1  SampleTime=1e-08
  Add : Subsystem
      mask Display: disp('NFP\nadd');
  Add1 : Subsystem
      mask Display: disp('NFP\nadd');
  Add2 : Subsystem
      mask Display: disp('NFP\nadd');
  Add3 : Subsystem
      mask Display: disp('NFP\nadd');
  Add4 : Subsystem
      mask Display: disp('NFP\nadd');
  Product1 : Subsystem
      mask Display: disp('NFP\nmul');
  Product10 : Subsystem
      mask Display: disp('NFP\nmul');
  Product11 : Subsystem
      mask Display: disp('NFP\nmul');
  Product2 : Subsystem
      mask Display: disp('NFP\nmul');
  Product3 : Subsystem
      mask Display: disp('NFP\nmul');
  Product31 : Subsystem
      mask Display: disp('NFP\nmul');
  Product4 : Subsystem
      mask Display: disp('NFP\nmul');
  Product5 : Subsystem
      mask Display: disp('NFP\nmul');
  Product6 : Subsystem
      mask Display: disp('NFP\nmul');
  Product7 : Subsystem
      mask Display: disp('NFP\nmul');
  Product8 : Subsystem
      mask Display: disp('NFP\nmul');
  Product9 : Subsystem
      mask Display: disp('NFP\nmul');
  Subtract1_stage2 : Subsystem
      mask Display: disp('NFP\nadd');
  Subtract1_stage3 : Subsystem
      mask Display: disp('NFP\nadd');
  Subtract2 : Subsystem
      mask Display: disp('NFP\nadd');
  Subtract3 : Subsystem
      mask Display: disp('NFP\nadd');
  Subtract_stage2 : Subsystem
      mask Display: disp('NFP\nadd');
  Subtract_stage3 : Subsystem
      mask Display: disp('NFP\nadd');
  delayMatch : Delay  DelayLength=double(18)  InitialCondition=0  SampleTime=1e-08
  delayMatch1 : Delay  DelayLength=double(18)  InitialCondition=0  SampleTime=1e-08
  delayMatch{2,10..11,13,16..31} (20 alike) : Delay  DelayLength=double(6)  InitialCondition=0  SampleTime=1e-08
  delayMatch{5..9,12,14..15} (8 alike) : Delay  DelayLength=double(12)  InitialCondition=0  SampleTime=1e-08
  delayMatch3 : Delay  DelayLength=double(24)  InitialCondition=0  SampleTime=1e-08
  delayMatch4 : Delay  DelayLength=double(24)  InitialCondition=0  SampleTime=1e-08
  id_16 : Outport  SampleTime=1e-08
  iq_16 : Outport  Port=2  SampleTime=1e-08
  ix_16 : Outport  Port=3  SampleTime=1e-08
  iy_16 : Outport  Port=4  SampleTime=1e-08
  wires:
  delayMatch14/1 -> Product1/1(In1)
  delayMatch22/1 -> Product4/1(In1)
  delayMatch26/1 -> Product8/1(In1)
  delayMatch30/1 -> Product10/1(In1)
  delayMatch11/1 -> Subtract_stage2/1(In1)
  delayMatch17/1 -> Subtract1_stage2/1(In1)
  delayMatch25/1 -> Subtract2/1(In1)
  delayMatch29/1 -> Subtract3/1(In1)
  delayMatch15/1 -> Add/2(In2)
  delayMatch12/1 -> Product31/2(In2)
  delayMatch27/1 -> Add3/2(In2)
  delayMatch31/1 -> Add4/2(In2)
  delayMatch19/1 -> Add2/1(In1)
  delayMatch20/1 -> Product6/1(In1)
  delayMatch13/1 -> Subtract_stage3/1(In1)
  delayMatch21/1 -> Subtract1_stage3/1(In1)
  Add/1(Out1) -> id_16/1
  Add1/1(Out1) -> iq_16/1
  Add2/1(Out1) -> Product6/2(In2)
  Add3/1(Out1) -> ix_16/1
  Add4/1(Out1) -> iy_16/1
  Product1/1(Out1) -> Add/1(In1)
  Product10/1(Out1) -> Add4/1(In1)
  Product11/1(Out1) -> Subtract3/2(In2)
  Product2/1(Out1) -> Subtract_stage2/2(In2)
  Product3/1(Out1) -> Product31/1(In1)
  Product31/1(Out1) -> Subtract_stage3/2(In2)
  Product4/1(Out1) -> Add1/1(In1)
  Product5/1(Out1) -> Subtract1_stage2/2(In2)
  Product6/1(Out1) -> Subtract1_stage3/2(In2)
  Product7/1(Out1) -> Add2/2(In2)
  Product8/1(Out1) -> Add3/1(In1)
  Product9/1(Out1) -> Subtract2/2(In2)
  Subtract_stage2/1(Out1) -> delayMatch13/1
  Subtract_stage3/1(Out1) -> Product1/2(In2)
  Subtract1_stage2/1(Out1) -> delayMatch21/1
  Subtract1_stage3/1(Out1) -> Product4/2(In2)
  Subtract2/1(Out1) -> Product8/2(In2)
  Subtract3/1(Out1) -> Product10/2(In2)
  delayMatch23/1 -> Add1/2(In2)
  delayMatch9/1 -> Product3/2(In2)
  delayMatch18/1 -> Product7/2(In2)
  delayMatch10/1 -> Product2/2(In2)
  delayMatch16/1 -> Product5/2(In2)
  delayMatch/1 -> delayMatch14/1
  delayMatch1/1 -> delayMatch15/1
  delayMatch24/1 -> Product9/2(In2)
  delayMatch2/1 -> delayMatch19/1
  delayMatch3/1 -> delayMatch22/1
  delayMatch4/1 -> delayMatch23/1
  delayMatch28/1 -> Product11/2(In2)
  delayMatch5/1 -> delayMatch26/1
  delayMatch6/1 -> delayMatch27/1
  delayMatch7/1 -> delayMatch30/1
  delayMatch8/1 -> delayMatch31/1
  SampleTime_div_Ld/1 -> delayMatch/1
  SampleTime_div_Lq/1 -> delayMatch3/1
  SampleTime_div_Lx/1 -> delayMatch5/1
  SampleTime_div_Ly/1 -> delayMatch7/1
  d_phase_voltage_per_switching_state/1 -> delayMatch11/1
  q_phase_voltage_per_switching_state/1 -> delayMatch17/1
  x_phase_voltage_per_switching_state/1 -> delayMatch25/1
  y_phase_voltage_per_switching_state/1 -> delayMatch29/1
  id_k/1 -> delayMatch1/1, Product7/1(In1), Product2/1(In1)
  iq_k/1 -> delayMatch4/1, Product5/1(In1), delayMatch12/1
  ix_k/1 -> delayMatch6/1, Product9/1(In1)
  iy_k/1 -> delayMatch8/1, Product11/1(In1)
  psiPM/1 -> delayMatch2/1
  Lq/1 -> delayMatch9/1
  Ld/1 -> delayMatch18/1
  Rs/1 -> delayMatch28/1, delayMatch24/1, delayMatch16/1, delayMatch10/1
  omega_el/1 -> Product3/1(In1), delayMatch20/1

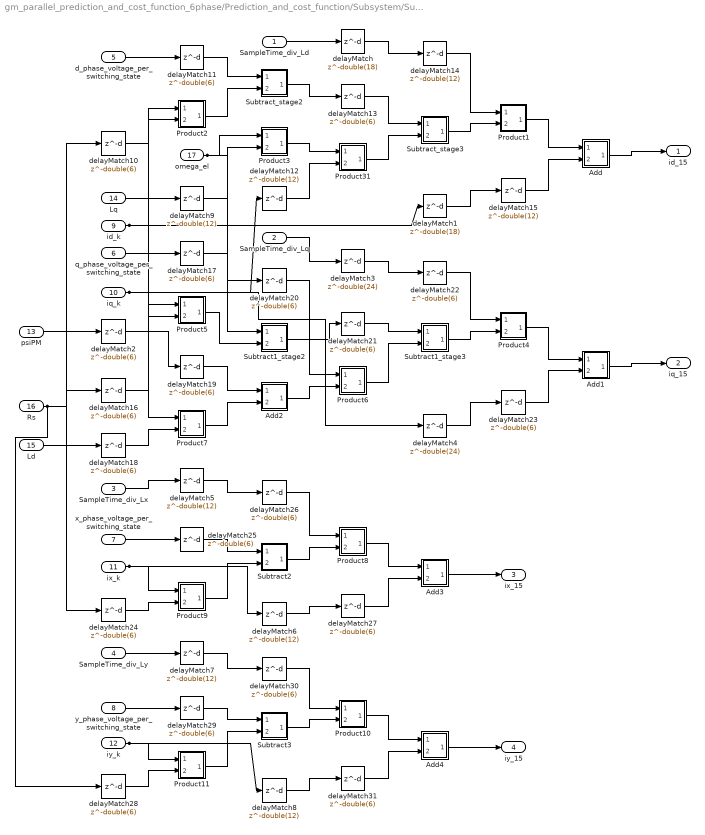
== system gm_parallel_prediction_and_cost_function_6phase/Prediction_and_cost_function/Subsystem/Subsystem1 ==
  SampleTime_div_Ld : Inport  OutDataTypeStr=single  PortDimensions=1  SampleTime=1e-08
  SampleTime_div_Lq : Inport  Port=2  OutDataTypeStr=single  PortDimensions=1  SampleTime=1e-08
  SampleTime_div_Lx : Inport  Port=3  OutDataTypeStr=single  PortDimensions=1  SampleTime=1e-08
  SampleTime_div_Ly : Inport  Port=4  OutDataTypeStr=single  PortDimensions=1  SampleTime=1e-08
  d_phase_voltage_per_switching_state : Inport  Port=5  OutDataTypeStr=single  PortDimensions=1  SampleTime=1e-08
  q_phase_voltage_per_switching_state : Inport  Port=6  OutDataTypeStr=single  PortDimensions=1  SampleTime=1e-08
  x_phase_voltage_per_switching_state : Inport  Port=7  OutDataTypeStr=single  PortDimensions=1  SampleTime=1e-08
  y_phase_voltage_per_switching_state : Inport  Port=8  OutDataTypeStr=single  PortDimensions=1  SampleTime=1e-08
  id_k : Inport  Port=9  OutDataTypeStr=single  PortDimensions=1  SampleTime=1e-08
  iq_k : Inport  Port=10  OutDataTypeStr=single  PortDimensions=1  SampleTime=1e-08
  ix_k : Inport  Port=11  OutDataTypeStr=single  PortDimensions=1  SampleTime=1e-08
  iy_k : Inport  Port=12  OutDataTypeStr=single  PortDimensions=1  SampleTime=1e-08
  psiPM : Inport  Port=13  OutDataTypeStr=single  PortDimensions=1  SampleTime=1e-08
  Lq : Inport  Port=14  OutDataTypeStr=single  PortDimensions=1  SampleTime=1e-08
  Ld : Inport  Port=15  OutDataTypeStr=single  PortDimensions=1  SampleTime=1e-08
  Rs : Inport  Port=16  OutDataTypeStr=single  PortDimensions=1  SampleTime=1e-08
  omega_el : Inport  Port=17  OutDataTypeStr=single  PortDimensions=1  SampleTime=1e-08
  Add : Subsystem
      mask Display: disp('NFP\nadd');
  Add1 : Subsystem
      mask Display: disp('NFP\nadd');
  Add2 : Subsystem
      mask Display: disp('NFP\nadd');
  Add3 : Subsystem
      mask Display: disp('NFP\nadd');
  Add4 : Subsystem
      mask Display: disp('NFP\nadd');
  Product1 : Subsystem
      mask Display: disp('NFP\nmul');
  Product10 : Subsystem
      mask Display: disp('NFP\nmul');
  Product11 : Subsystem
      mask Display: disp('NFP\nmul');
  Product2 : Subsystem
      mask Display: disp('NFP\nmul');
  Product3 : Subsystem
      mask Display: disp('NFP\nmul');
  Product31 : Subsystem
      mask Display: disp('NFP\nmul');
  Product4 : Subsystem
      mask Display: disp('NFP\nmul');
  Product5 : Subsystem
      mask Display: disp('NFP\nmul');
  Product6 : Subsystem
      mask Display: disp('NFP\nmul');
  Product7 : Subsystem
      mask Display: disp('NFP\nmul');
  Product8 : Subsystem
      mask Display: disp('NFP\nmul');
  Product9 : Subsystem
      mask Display: disp('NFP\nmul');
  Subtract1_stage2 : Subsystem
      mask Display: disp('NFP\nadd');
  Subtract1_stage3 : Subsystem
      mask Display: disp('NFP\nadd');
  Subtract2 : Subsystem
      mask Display: disp('NFP\nadd');
  Subtract3 : Subsystem
      mask Display: disp('NFP\nadd');
  Subtract_stage2 : Subsystem
      mask Display: disp('NFP\nadd');
  Subtract_stage3 : Subsystem
      mask Display: disp('NFP\nadd');
  delayMatch : Delay  DelayLength=double(18)  InitialCondition=0  SampleTime=1e-08
  delayMatch1 : Delay  DelayLength=double(18)  InitialCondition=0  SampleTime=1e-08
  delayMatch{2,10..11,13,16..31} (20 alike) : Delay  DelayLength=double(6)  InitialCondition=0  SampleTime=1e-08
  delayMatch{5..9,12,14..15} (8 alike) : Delay  DelayLength=double(12)  InitialCondition=0  SampleTime=1e-08
  delayMatch3 : Delay  DelayLength=double(24)  InitialCondition=0  SampleTime=1e-08
  delayMatch4 : Delay  DelayLength=double(24)  InitialCondition=0  SampleTime=1e-08
  id_15 : Outport  SampleTime=1e-08
  iq_15 : Outport  Port=2  SampleTime=1e-08
  ix_15 : Outport  Port=3  SampleTime=1e-08
  iy_15 : Outport  Port=4  SampleTime=1e-08
  wires:
  delayMatch13/1 -> Subtract_stage3/1(In1)
  delayMatch21/1 -> Subtract1_stage3/1(In1)
  delayMatch14/1 -> Product1/1(In1)
  delayMatch22/1 -> Product4/1(In1)
  delayMatch26/1 -> Product8/1(In1)
  delayMatch30/1 -> Product10/1(In1)
  delayMatch11/1 -> Subtract_stage2/1(In1)
  delayMatch17/1 -> Subtract1_stage2/1(In1)
  delayMatch25/1 -> Subtract2/1(In1)
  delayMatch29/1 -> Subtract3/1(In1)
  delayMatch15/1 -> Add/2(In2)
  delayMatch12/1 -> Product31/2(In2)
  delayMatch27/1 -> Add3/2(In2)
  delayMatch31/1 -> Add4/2(In2)
  delayMatch19/1 -> Add2/1(In1)
  delayMatch20/1 -> Product6/1(In1)
  Add/1(Out1) -> id_15/1
  Add1/1(Out1) -> iq_15/1
  Add2/1(Out1) -> Product6/2(In2)
  Add3/1(Out1) -> ix_15/1
  Add4/1(Out1) -> iy_15/1
  Product1/1(Out1) -> Add/1(In1)
  Product10/1(Out1) -> Add4/1(In1)
  Product11/1(Out1) -> Subtract3/2(In2)
  Product2/1(Out1) -> Subtract_stage2/2(In2)
  Product3/1(Out1) -> Product31/1(In1)
  Product31/1(Out1) -> Subtract_stage3/2(In2)
  Product4/1(Out1) -> Add1/1(In1)
  Product5/1(Out1) -> Subtract1_stage2/2(In2)
  Product6/1(Out1) -> Subtract1_stage3/2(In2)
  Product7/1(Out1) -> Add2/2(In2)
  Product8/1(Out1) -> Add3/1(In1)
  Product9/1(Out1) -> Subtract2/2(In2)
  Subtract_stage2/1(Out1) -> delayMatch13/1
  Subtract_stage3/1(Out1) -> Product1/2(In2)
  Subtract1_stage2/1(Out1) -> delayMatch21/1
  Subtract1_stage3/1(Out1) -> Product4/2(In2)
  Subtract2/1(Out1) -> Product8/2(In2)
  Subtract3/1(Out1) -> Product10/2(In2)
  delayMatch23/1 -> Add1/2(In2)
  delayMatch9/1 -> Product3/2(In2)
  delayMatch18/1 -> Product7/2(In2)
  delayMatch10/1 -> Product2/2(In2)
  delayMatch16/1 -> Product5/2(In2)
  delayMatch/1 -> delayMatch14/1
  delayMatch1/1 -> delayMatch15/1
  delayMatch24/1 -> Product9/2(In2)
  delayMatch2/1 -> delayMatch19/1
  delayMatch3/1 -> delayMatch22/1
  delayMatch4/1 -> delayMatch23/1
  delayMatch28/1 -> Product11/2(In2)
  delayMatch5/1 -> delayMatch26/1
  delayMatch6/1 -> delayMatch27/1
  delayMatch7/1 -> delayMatch30/1
  delayMatch8/1 -> delayMatch31/1
  SampleTime_div_Ld/1 -> delayMatch/1
  SampleTime_div_Lq/1 -> delayMatch3/1
  SampleTime_div_Lx/1 -> delayMatch5/1
  SampleTime_div_Ly/1 -> delayMatch7/1
  d_phase_voltage_per_switching_state/1 -> delayMatch11/1
  q_phase_voltage_per_switching_state/1 -> delayMatch17/1
  x_phase_voltage_per_switching_state/1 -> delayMatch25/1
  y_phase_voltage_per_switching_state/1 -> delayMatch29/1
  id_k/1 -> delayMatch1/1, Product7/1(In1), Product2/1(In1)
  iq_k/1 -> delayMatch4/1, Product5/1(In1), delayMatch12/1
  ix_k/1 -> delayMatch6/1, Product9/1(In1)
  iy_k/1 -> delayMatch8/1, Product11/1(In1)
  psiPM/1 -> delayMatch2/1
  Lq/1 -> delayMatch9/1
  Ld/1 -> delayMatch18/1
  Rs/1 -> delayMatch28/1, delayMatch24/1, delayMatch16/1, delayMatch10/1
  omega_el/1 -> Product3/1(In1), delayMatch20/1
